simulink model "slb_counter_pulgen"  (R2015b)
settings: Solver=FixedStepDiscrete  SolverMode=SingleTasking  StartTime=0.0  StopTime=2000  RelTol=1e-3
libraries: simulink x5, hdlsllib x2
settings Model: Creator=at-mt  LastModifiedBy=amatsumo
settings DataIOCC: SaveFormat=Array  SignalLoggingSaveFormat=ModelDataLogs  SaveOutput=off  SignalLogging=off  SaveTime=off
settings OptimizationCC: BlockReduction=off  ConditionallyExecuteInputs=off  DefaultParameterBehavior=Inlined  ExpressionDepthLimit=2147483647
settings DebuggingCC: AlgebraicLoopMsg=error  UnderspecifiedInitializationDetection=Classic  MergeDetectMultiDrivingBlocksExec=none  SolverPrmCheckMsg=warning  SingleTaskRateTransMsg=error  FcnCallInpInsideContextMsg=UseLocalSettings  StateNameClashWarn=warning
settings HardwareCC: ProdBitPerPointer=32  ProdLargestAtomicFloat=None  ProdIntDivRoundTo=Undefined  ProdEndianess=Unspecified  ProdWordSize=32  ProdHWDeviceType=ASIC/FPGA->ASIC/FPGA  ProdEqTarget=off
settings SFSimCC: SFSimEcho=off
settings GRTTargetCC: GeneratePreprocessorConditionals=Disable all  CombineOutputUpdateFcns=off  GRTInterface=on
settings ConfigComp: CovModelRefEnable=Off  CovSFcnEnable=off

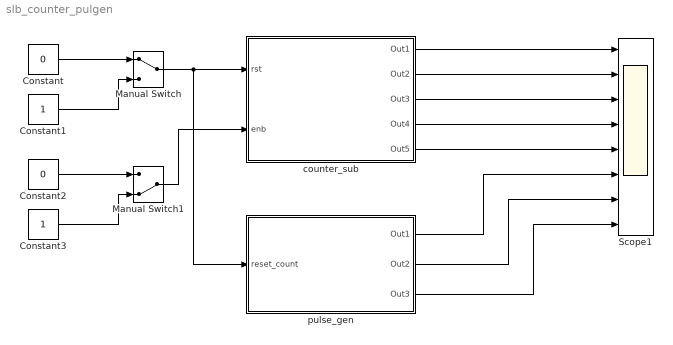
== system slb_counter_pulgen ==
  Constant : Constant  Value=0  OutDataTypeStr=boolean  SampleTime=1
  Constant1 : Constant  OutDataTypeStr=boolean  SampleTime=1
  Constant2 : Constant  Value=0  OutDataTypeStr=boolean  SampleTime=1
  Constant3 : Constant  OutDataTypeStr=boolean  SampleTime=1
  Manual Switch : ManualSwitch
  Manual Switch1 : ManualSwitch  CurrentSetting=0
  Scope1 : Scope  NumInputPorts=8
  counter_sub : Subsystem
  pulse_gen : Subsystem
  wires:
  Constant/1 -> Manual Switch/1
  Constant1/1 -> Manual Switch/2
  counter_sub/3(Out3) -> Scope1/3
  counter_sub/4(Out4) -> Scope1/4
  counter_sub/1(Out1) -> Scope1/1
  counter_sub/2(Out2) -> Scope1/2
  counter_sub/5(Out5) -> Scope1/5
  Manual Switch/1 -> pulse_gen/1(reset_count), counter_sub/1(rst)
  pulse_gen/1(Out1) -> Scope1/6
  pulse_gen/2(Out2) -> Scope1/7
  pulse_gen/3(Out3) -> Scope1/8
  Constant2/1 -> Manual Switch1/1
  Constant3/1 -> Manual Switch1/2
  Manual Switch1/1 -> counter_sub/2(enb)

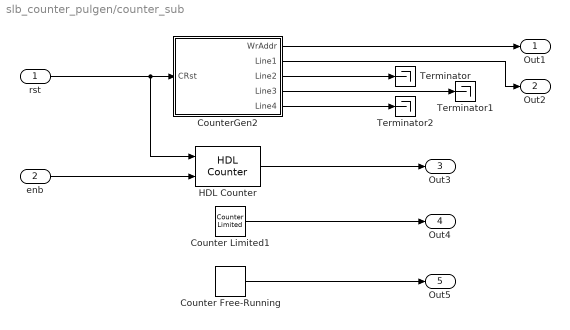
== system slb_counter_pulgen/counter_sub ==
  rst : Inport
  enb : Inport  Port=2
  Counter Free-Running : simulink/Sources/Counter Free-Running  NumBits=8  tsamp=-1
  Counter Limited1 : simulink/Sources/Counter Limited  uplimit=240-1  tsamp=1
  CounterGen2 : MATLAB Function  TreatAsAtomicUnit=on
  HDL Counter : hdlsllib/HDL Operations/HDL Counter  CountType=Count limited  CountInit=240-1  CountStep=-1  CountMax=0  CountFromType=Initial value  CountFrom=240-1  CountResetPort=on  CountLoadPort=off  CountEnbPort=on  CountDirPort=off  CountDataType=Unsigned  CountWordLen=8  CountFracLen=0  CountSampTime=1
  Terminator : Terminator
  Terminator1 : Terminator
  Terminator2 : Terminator
  Out1 : Outport
  Out2 : Outport  Port=2
  Out3 : Outport  Port=3
  Out4 : Outport  Port=4
  Out5 : Outport  Port=5
  wires:
  rst/1 -> HDL Counter/1, CounterGen2/1(CRst)
  CounterGen2/1(WrAddr) -> Out1/1
  CounterGen2/2(Line1) -> Out2/1
  CounterGen2/3(Line2) -> Terminator/1
  CounterGen2/4(Line3) -> Terminator1/1
  CounterGen2/5(Line4) -> Terminator2/1
  HDL Counter/1 -> Out3/1
  Counter Limited1/1 -> Out4/1
  Counter Free-Running/1 -> Out5/1
  enb/1 -> HDL Counter/2

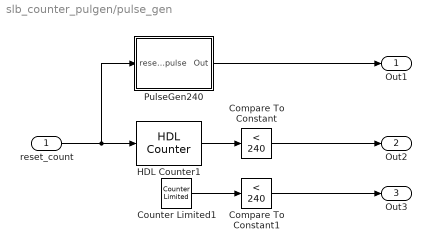
== system slb_counter_pulgen/pulse_gen ==
  reset_count : Inport
  Compare To Constant : simulink/Logic and Bit Operations/Compare To Constant  relop=<  const=240  OutDataTypeStr=uint8  ZeroCross=off
  Compare To Constant1 : simulink/Logic and Bit Operations/Compare To Constant  relop=<  const=240  OutDataTypeStr=uint8  ZeroCross=off
  Counter Limited1 : simulink/Sources/Counter Limited  uplimit=240*2-1  tsamp=1
  HDL Counter1 : hdlsllib/HDL Operations/HDL Counter  CountType=Count limited  CountInit=0  CountStep=1  CountMax=240*2-1  CountFromType=Initial value  CountFrom=0  CountResetPort=on  CountLoadPort=off  CountEnbPort=off  CountDirPort=off  CountDataType=Unsigned  CountWordLen=10  CountFracLen=0  CountSampTime=1
  PulseGen240 : MATLAB Function  TreatAsAtomicUnit=on
  Out1 : Outport
  Out2 : Outport  Port=2
  Out3 : Outport  Port=3
  wires:
  Counter Limited1/1 -> Compare To Constant1/1
  HDL Counter1/1 -> Compare To Constant/1
  PulseGen240/1(Out) -> Out1/1
  reset_count/1 -> HDL Counter1/1, PulseGen240/1(reset_pulse)
  Compare To Constant/1 -> Out2/1
  Compare To Constant1/1 -> Out3/1

== matlab function slb_counter_pulgen/counter_sub/CounterGen2 ==
  settings: updateMethod=DISCRETE  sampleTime=1
  data: WrAddr output; Line1 output; Line2 output; Line3 output; CRst input boolean; Line4 output
function [WrAddr,Line1,Line2,Line3,Line4] = counter(CRst)
% This block supports the Embedded MATLAB subset.
% See the help menu for details. 

% Parameters
DelayNum=240;
UpperLim = DelayNum*4;

Type_nt = numerictype(0,ceil(log2(UpperLim)),0);
Type_fm = fimath('OverflowMode', 'wrap', 'RoundMode', 'floor');

Line1Lim = fi(UpperLim-DelayNum,Type_nt, Type_fm);
Line2Lim = fi(UpperLim-(DelayNum*2),Type_nt, Type_fm);
Line3Lim = fi(UpperLim-(DelayNum*3),Type_nt, Type_fm);
Line4Lim = fi(UpperLim-(DelayNum*4),Type_nt, Type_fm);


persistent CountTemp

if isempty(CountTemp)
	CountTemp = fi(0,Type_nt, Type_fm);
end

% Output Count Down Signal
if ((CountTemp > 0)&&(CRst == 0))
	Temp = CountTemp-fi(1,Type_nt, Type_fm);
	CountTemp = fi(Temp, Type_nt, Type_fm);
else
	CountTemp = fi(UpperLim-1,Type_nt, Type_fm);
end

WrAddr = CountTemp;
if CountTemp >= Line1Lim
	Temp1 = fi(CountTemp-UpperLim+DelayNum,Type_nt, Type_fm);
	Line1 = Temp1;
else
	Temp1 = fi(CountTemp+DelayNum,Type_nt, Type_fm);
	Line1 = Temp1;
end

if CountTemp >= Line2Lim
	Temp2 = fi(CountTemp-UpperLim+(DelayNum*2),Type_nt, Type_fm);
	Line2 = Temp2;
else
	Temp2 = fi(CountTemp+(DelayNum*2),Type_nt, Type_fm);
	Line2 = Temp2;
end

if CountTemp >= Line3Lim
	Temp3 = fi(CountTemp-UpperLim+(DelayNum*3),Type_nt, Type_fm);
	Line3 = Temp3;
else
	Temp3 = fi(CountTemp+(DelayNum*3),Type_nt, Type_fm);
	Line3 = Temp3;
end

if CountTemp >= Line4Lim
	Temp4 = fi(CountTemp-UpperLim+(DelayNum*4),Type_nt, Type_fm);
	Line4 = Temp4;
else
	Temp4 = fi(CountTemp+(DelayNum*4),Type_nt, Type_fm);
	Line4 = Temp4;
end

== matlab function slb_counter_pulgen/pulse_gen/PulseGen240 ==
  settings: updateMethod=DISCRETE  sampleTime=1
  data: Out output boolean; reset_pulse input boolean
function Out = counter(reset_pulse)
% This block supports the Embedded MATLAB subset.
% See the help menu for details. 

% Parameters
Cycle = 240*2;
PulseWidth = 240;
PhaseOffset = 0;

Type_nt = numerictype(0,10,0);
Type_nt1 = numerictype(0,11,0);
Type_fm = fimath('OverflowMode', 'wrap', 'RoundMode', 'floor');

persistent CountTemp Temp

if isempty(CountTemp)
	CountTemp = fi(0,Type_nt, Type_fm);
	Temp = fi(0,Type_nt, Type_fm);
end

% Output Pulse Signal
if (CountTemp >= PhaseOffset)&&(CountTemp < PulseWidth+PhaseOffset)
	Out = logical(1);
else
	Out = logical(0);
end
if (CountTemp >= Cycle-1)||reset_pulse;
	CountTemp = fi(0,Type_nt, Type_fm);
else
	Temp = fi(CountTemp+1,Type_nt, Type_fm);
	CountTemp = fi(Temp, Type_nt, Type_fm);
end
